simulink model "a_LS_model2"  (R2023b)
settings: Solver=VariableStepAuto  StartTime=0.0  StopTime=3  RelTol=1e-3
PreLoadFcn:
  | %% Model component value calculations with holder values.
  | clear;
  | disp('PreLoaded holder values run model to apply entered T&S values ')
  | 
  | Re = [1, 1]; % The DC resistance of the Voice coil [ohm].
  | 
  | Le = [1, 1]; % The voice coil inductance [H]
  | 
  | Mms = [1, 1]; % Mass of the coil and diaphragm [Kg]
  | 
  | Sd = [1, 1] * 1e-4; % Area of diaphragm [m^2]
  | 
  | Bl = [1, 1]; % The product of magnetic flux density i.e., Force Factor
  | 
  | Vb = [1, 1];
  | 
  | fs = [1, 1];
  | 
  | Qes = [1, 1];
  | 
  | Qms = [1, 1];
  | 
  | Qts = [1, 1];
  | 
  | SweepStart_W_S = 1;
  | SweepEnd_W_S = 1;
  | SweepDuration_W_S = 1;
  | FS = 44100;
  | Qb = 0.707; % Total quality factor
  | 
  | % Constants
  | c = 340; % Speed of sound in m/s
  | rho = 1.2; % Density of air [kg/m^3]
  | r=1; % Distance for farfield calculations
  | wOffset = 0; % Driver offset for fafield calculations
  | tOffset = 0;
  | dt=1/FS; % Time step
  | for n = 1:2
  |     alpha(n) = (Qb^2 - Qts(n)^2) / Qts(n)^2;
  |     Rms(n) = (2 * pi * fs(n) * Mms(n)) / Qms(n);
  |     Cms(n) = 1 / (4 * pi^2 * fs(n)^2 * Mms(n));
  |     Vas(n) = rho * c * Sd(n)^2 * Cms(n);
  | end
  | 
  | QB = sqrt(alpha(1) + 1) * Qts; % Electroacoustics Lecture 4 page 21
  | 
  | for n = 1:2
  |     r = 0.1;
  |     Cab(n) = Vb(n) / (rho * c^2); % Box volume acoustic compliance
  |     a(n) = sqrt(Sd(n) / pi);
  |     a(n) = 0.85;
  | 
  |     % Zc(n) = ((rho * c) / Sd(n)) * c; % from grain42n
  |     Mad(n) = (8 * rho) / (5 * (pi^2) * a(n)); % Mad (acoustic mass)
  |     Mar(n) = rho * ((a(n) * r) / Sd(n)); % from grain42n
  |     Mad(n) = Mar(n);
  | 
  |     Ras(n) = (rho * c) / (pi * (a(n)^2)); % Ras (acoustic resistance), Beranek page 820/ grain42-page 19
  |     Lem(n) = Bl(n)^2 * Cms(n); % Lem (driver's equivalent inductance)
  |     Rem(n) = Bl(n)^2 / Rms(n); % Rem (driver's equivalent mechanical resistance)
  | ... (+17 lines)
StartFcn:
  | %% Model Component Value Calculations
  | close all;
  | 
  | disp('Thiele and Small Parameters Loaded');
  | disp('Loudspeaker Simulation Running...');
  | 
  | % Load parameters from the mask
  | Box_plot_flag = get_param('a_LS_model/T&S Values', 'Box_Plot');
  | Combo_plot_flag = get_param('a_LS_model/T&S Values', 'DSP_Plot');
  | wImpedance_plot_flag = get_param('a_LS_model/T&S Values', 'wImpedance_Plot');
  | tImpedance_plot_flag = get_param('a_LS_model/T&S Values', 'tImpedance_Plot');
  | Re = [str2double(get_param('a_LS_model/T&S Values', 'W_Re')), str2double(get_param('a_LS_model/T&S Values', 'T_Re'))]; % DC resistance of the Voice coil [ohm].
  | Le = [str2double(get_param('a_LS_model/T&S Values', 'W_Le')), str2double(get_param('a_LS_model/T&S Values', 'T_Le'))] * 1e-3; % Voice coil inductance [H]
  | Mms = [str2double(get_param('a_LS_model/T&S Values', 'W_Mms')), str2double(get_param('a_LS_model/T&S Values', 'T_Mms'))] * 1e-3; % Mass of the coil and diaphragm [Kg]
  | Sd = [str2double(get_param('a_LS_model/T&S Values', 'W_Sd')), str2double(get_param('a_LS_model/T&S Values', 'T_Sd'))] * 1e-4; % Area of diaphragm [m^2]
  | Bl = [str2double(get_param('a_LS_model/T&S Values', 'W_Bl')), str2double(get_param('a_LS_model/T&S Values', 'T_Bl'))]; % Magnetic flux density product (Force Factor)
  | Vb = [str2double(get_param('a_LS_model/T&S Values', 'Vb')), str2double(get_param('a_LS_model/T&S Values', 'Vb'))];
  | fs = [str2double(get_param('a_LS_model/T&S Values', 'W_fs')), str2double(get_param('a_LS_model/T&S Values', 'T_fs'))];
  | Cms = [str2double(get_param('a_LS_model/T&S Values', 'W_Cms')), str2double(get_param('a_LS_model/T&S Values', 'W_Cms'))];
  | Qes = [str2double(get_param('a_LS_model/T&S Values', 'W_Qes')), str2double(get_param('a_LS_model/T&S Values', 'T_Qes'))];
  | Qms = [str2double(get_param('a_LS_model/T&S Values', 'W_Qms')), str2double(get_param('a_LS_model/T&S Values', 'T_Qms'))];
  | Qts = [str2double(get_param('a_LS_model/T&S Values', 'W_Qts')), str2double(get_param('a_LS_model/T&S Values', 'T_Qts'))];
  | 
  | % Load additional parameters
  | SweepStart_W_S = str2double(get_param('a_LS_model/Subsystem4', 'SweepStart'));
  | SweepEnd_W_S = str2double(get_param('a_LS_model/Subsystem4', 'SweepStop'));
  | SweepDuration_W_S = str2double(get_param('a_LS_model/Subsystem4', 'SweepTime'));
  | 
  | figSaveFolder = get_param('a_LS_model/Teensy Script', 'figSaveFolder');
  | 
  | FS = 44100;
  | 
  | % Constants
  | c = 343; % Speed of sound in m/s
  | rho = 1.2; % Density of air [kg/m^3]
  | wOffset = str2double(get_param('a_LS_model/Subsystem1', 'distW'));
  | tOffset = str2double(get_param('a_LS_model/Subsystem1', 'distT'));
  | dt=1/FS; %time step
  | 
  | Vas(1) = rho * c * Sd(1)^2 * Cms(1);
  | 
  | for n = 1:2
  |     if n == 1
  |      fsBx = fs(1) *(Vas(1)/Vb(1)+1)^(1/2);
  |      aV = Vas(1) / Vb(1);
  |      Qb(n) = Qts(n) * sqrt(1 + aV);
  |      Rms(n) = (2 * pi * fs(n) * Mms(n)) / Qms(n);
  |      Cms(n) = 1 / ((2 * pi * fs(n))^2 * Mms(n));
  |      CmsBx = 1 / ((2 * pi * fsBx)^2 * Mms(n));
  |      QmsBx =  (2*pi*fsBx*Mms(1))/Rms(1);
  |      RmsBx = (2 * pi * fsBx * Mms(n)) / (QmsBx);
  |     elseif n == 2
  | 
  |      Cms(n) = 1 / ((2 * pi * fs(n))^2 * Mms(n));
  |      Rms(n) = (2 * pi * fs(n) * Mms(n)) / Qms(n);
  |      Vas(n) = rho * c * Sd(n)^2 * Cms(n);
  | 
  |     end
  |    alpha(n) = (Qb^2 - Qts(n)^2) / Qts(n)^2;
  | 
  | ... (+443 lines)
StopFcn:
  | disp('Simulation Ended')
undefined symbols (not defined in the file): Ced, Cem, Cer, Leb, Lem, Rem
libraries: fl_lib x29, nesl_utility x12, dspsrcs4 x1
(part 2 of 2)

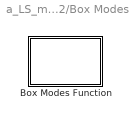
== system a_LS_model2/Box Modes ==
  Box Modes Function : MATLAB Function  TreatAsAtomicUnit=on

== system a_LS_model2/Bypass ==

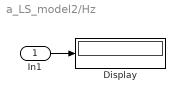
== system a_LS_model2/Hz ==
  In1 : Inport
  Display : Display
  wires:
  In1/1 -> Display/1

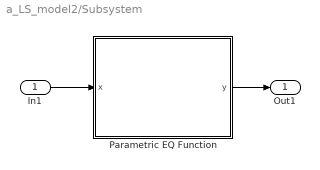
== system a_LS_model2/Subsystem ==
  In1 : Inport
  Parametric EQ Function : MATLAB Function  TreatAsAtomicUnit=on
  Out1 : Outport
  wires:
  In1/1 -> Parametric EQ Function/1(x)
  Parametric EQ Function/1(y) -> Out1/1

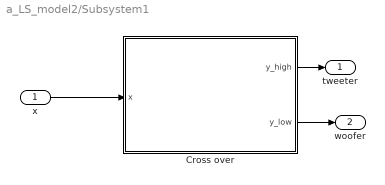
== system a_LS_model2/Subsystem1 ==
  x : Inport
  Cross over : MATLAB Function  TreatAsAtomicUnit=on
  tweeter : Outport
  woofer : Outport  Port=2
  wires:
  x/1 -> Cross over/1(x)
  Cross over/1(y_high) -> tweeter/1
  Cross over/2(y_low) -> woofer/1

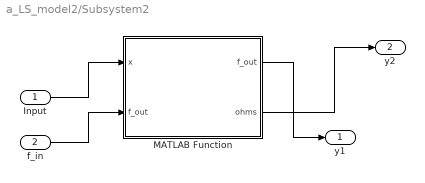
== system a_LS_model2/Subsystem2 ==
  Input : Inport
  f_in : Inport  Port=2
  MATLAB Function : MATLAB Function  TreatAsAtomicUnit=on
  y1 : Outport
  y2 : Outport  Port=2
  wires:
  MATLAB Function/1(f_out) -> y1/1
  Input/1 -> MATLAB Function/1(x)
  MATLAB Function/2(ohms) -> y2/1
  f_in/1 -> MATLAB Function/2("f_out ")

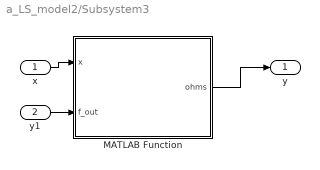
== system a_LS_model2/Subsystem3 ==
  x : Inport
  y1 : Inport  Port=2
  MATLAB Function : MATLAB Function  TreatAsAtomicUnit=on
  y : Outport
  wires:
  x/1 -> MATLAB Function/1(x)
  MATLAB Function/1(ohms) -> y/1
  y1/1 -> MATLAB Function/2(f_out)

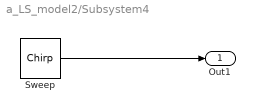
== system a_LS_model2/Subsystem4 ==
  Sweep : dspsrcs4/Chirp  sweep=Logarithmic  mode=Unidirectional  f0=SweepStart  f1=SweepStop  t1=SweepTime  Tsweep=SweepTime  phase=0  Ts=1/FS  spf=1024  datatype=Double  OutputFrames=off
  Out1 : Outport
  wires:
  Sweep/1 -> Out1/1

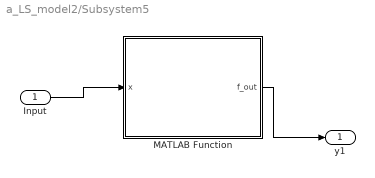
== system a_LS_model2/Subsystem5 ==
  Input : Inport
  MATLAB Function : MATLAB Function  TreatAsAtomicUnit=on
  y1 : Outport
  wires:
  MATLAB Function/1(f_out) -> y1/1
  Input/1 -> MATLAB Function/1(x)

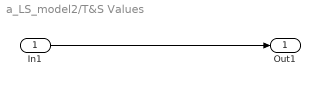
== system a_LS_model2/T&S Values ==
  In1 : Inport
  Out1 : Outport
  wires:
  In1/1 -> Out1/1

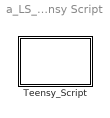
== system a_LS_model2/Teensy Script ==
  Teensy_Script : MATLAB Function  TreatAsAtomicUnit=on

== matlab function a_LS_model2/Subsystem1/Cross over ==
  data: x input; y_high output; y_low output
%% Linkwitz and Riley Crossover function that recieves user parameters from Simulink mask

function [y_high,y_low]= crossover(x)

persistent zi_low_1 % Persistent filter states held over for next block
persistent zi_low_2

persistent zi_high_1
persistent zi_high_2



persistent flagBaseAssign             % flags for parts of code that only need to be run once to improve code efficiency



persistent frontPadT
persistent frontPadW
persistent delayBufferT
persistent delayBufferW


if isempty(flagBaseAssign)

    flagBaseAssign=1;

end


%wSamples=double(0);
%tSamples=double(0);
coder.extrinsic('get_param') %coder.entrinsic allows for functions to be surported in simulink that would otherwise not be
coder.extrinsic('xticks')
coder.extrinsic('xticklabels')
coder.extrinsic("assignin")
coder.extrinsic("evalin")
coder.extrinsic("sgtitle")
coder.extrinsic("cat")
coder.extrinsic("exist")
coder.extrinsic("mkdir")
coder.extrinsic("fullfile")
coder.extrinsic("mexFilter")




y_low =zeros(length(x),1);
y_high=zeros(length(x),1);


%Getting user input from mask

persistent tDistance wDistance G_T G_W filterOrder delayInfo B_low A_low B_high A_high plotFlag bypass fs...
    tweeterGain_dB wooferGain_dB

if isempty (tDistance)
    plotFlag = get_param('a_LS_model/Subsystem1', 'response');
    bypass = get_param('a_LS_model/Bypass', 'bypass');
    fs=44100;
    tDistance=double(0);
    tDistance = str2double(get_param('a_LS_model/Subsystem1', 'distT'));
    wDistance=double(0);
    wDistance = str2double(get_param('a_LS_model/Subsystem1', 'distW'));
    

    G_T = str2double(get_param('a_LS_model/Subsystem1', 'G_T'));
    G_W = str2double(get_param('a_LS_model/Subsystem1', 'G_W'));
    filterOrder = get_param('a_LS_model/Subsystem1', 'filter_order');
    delayInfo = get_param('a_LS_model/Subsystem1', 'delay');
    tweeterGain_dB = (10^(G_T/20));
    wooferGain_dB = (10^(G_W/20));

    fc = str2double(get_param('a_LS_model/Subsystem1', 'fc'));


    w=double(0);

    w =fc/(fs/2);



    if strcmp(filterOrder,'8th')

        butterOrder=4;

    elseif strcmp(filterOrder,'4th')

        butterOrder=2;

    else

        butterOrder=1;
    end



    [B_low, A_low]= butter(butterOrder, w, "low");

    [B_high, A_high]= butter(butterOrder, w, "high");



    assignin('base', 'B_Low_shel', B_low); % Assign to base for use in teensy script writing also speeds code as can be read rather than calulated for every block but first.
    assignin('base', 'A_Low_shel', A_low);

    assignin('base', 'B_High_shel', B_high);
    assignin('base', 'A_High_shel', A_high);





end


%%%%%%%%%%%%%%%%%%%%%%%%%%%%%%%%%%%%%%%%%%%%%%%%%%%%%%%%%%%%%%%%%%%%%%
%% Low pass


x_low=x;

if isempty (zi_low_1)
    zi_low_1=zeros(5,1);
    zi_low_2=zeros(5,1);


    zi_high_1=zeros(5,1);
    zi_high_2=zeros(5,1);

end




[y_low, zi_low_1]=mexFilter(B_low, A_low,x_low, zi_low_1);


x_low =y_low;

[y_low, zi_low_2]=mexFilter(B_low, A_low, x_low, zi_low_2);










%%%%%%%%%%%%%%%%%%%%%%%%%%%%%%%%%%%%%%%%%%%%%%%%%%%%%%%%%%%%%%%
%% High pass


x_high=x;



[y_high, zi_high_1]=mexFilter(B_high,A_high,x_high,zi_high_1);

x_high=y_high;


[y_high, zi_high_2]=mexFilter(B_high,A_high,x_high,zi_high_2);



y_high=y_high * tweeterGain_dB;
y_low=y_low * wooferGain_dB;


y_checkLow=y_low;   %%For delay debugging
y_checkHigh=y_high;


%% Plotting

if strcmp(plotFlag,'on')
    figure(2)

    [H_high, ~]=freqz(B_high,A_high);
    [H_low, w]=freqz(B_low,A_low);


    f=w/(2*pi)*fs;

    H_high_2=H_high.*H_high;

    H_low_2=H_low.*H_low;


    set(gcf, 'Position', [100, 100, 800, 600]);

    [H_high, ~]=freqz(B_high,A_high);
    [H_low, w]=freqz(B_low,A_low);


    f=w/(2*pi)*fs;

    H_high_2=H_high.*H_high;

    H_low_2=H_low.*H_low;



    subplot(3,1,1)
    semilogx(f, mag2db(abs(H_high_2)),'b-','DisplayName', 'Second Cascade');
    hold on
    semilogx(f, mag2db(abs(H_high)),'g-', 'DisplayName', 'First Cascade');
    hold off
    xlabel('Frequency (Hz)')
    ylabel('Magnitude (dB)')
    title('Magnitude Response High Pass')
    ylim([-14 14])
    xlim([min(f) max(f)])

    xticks([20 50 100 200 500 1000 2000 5000 10000 20000]);
    xticklabels({'20','50','100','200','500','1000','2000','5000','10000','20000'});
    legend('show', 'Location', 'best');
    subplot(3,1,2)
    semilogx(f, mag2db(abs(H_low_2)),'b-','DisplayName', 'Second Cascade');
    hold on
    semilogx(f, mag2db(abs(H_low)),'g-','DisplayName', 'First Cascade');
    hold off
    xlabel('Frequency (Hz)')
    ylabel('Magnitude (dB)')
    title('Magnitude Response Low pass')
    ylim([-14 14])
    xlim([min(f) max(f)])

    xticks([20 50 100 200 500 1000 2000 5000 10000 20000]);
    xticklabels({'20','50','100','200','500','1000','2000','5000','10000','20000'});
    legend('show', 'Location', 'best');
    subplot(3,1,3)
    semilogx(f, mag2db(abs(H_low_2)),'r--','DisplayName', 'Low Pass');
    hold on
    semilogx(f, mag2db(abs(H_high_2)),'r-','DisplayName', 'High Pass');
    legend('show', 'Location', 'best');
    if double(length(B_low))==2

        H_low_2_inverted=H_low_2.*-1;
        semilogx(f, mag2db(abs(H_high_2+H_low_2_inverted)),'b-','DisplayName', 'Combined Response');


        hold off
        xlabel('Frequency (Hz)')
        ylabel('Magnitude (dB)')
        title('Magnitude Response Linkwitz-Riley 2nd Order')

    elseif double(length(B_low))==3

        semilogx(f, mag2db(abs(H_high_2+H_low_2)),'b-','DisplayName', 'Combined Response');


        hold off
        xlabel('Frequency (Hz)')
        ylabel('Magnitude (dB)')
        title('Magnitude Response Linkwitz-Riley 4th Order')


    else

        semilogx(f, mag2db(abs(H_high_2+H_low_2)),'b-','DisplayName', 'Combined Response');


        hold off
        xlabel('Frequency (Hz)')
        ylabel('Magnitude (dB)')
        title('Magnitude Response Linkwitz-Riley 8th Order')

    end


    ylim([-14 14])
    xlim([min(f) max(f)])

    xticks([20 50 100 200 500 1000 2000 5000 10000 20000]);
    xticklabels({'20','50','100','200','500','1000','2000','5000','10000','20000'});

    if strcmp(filterOrder,'4th')

        sgtitle('Linkwitz-Riley 4th Order Crossover');

    elseif strcmp(filterOrder,'8th')

        sgtitle('Linkwitz-Riley 8th Order Crossover');

    else

        sgtitle('Linkwitz-Riley 2nd Order Crossover');

    end
    if strcmp(get_param('a_LS_model/Teensy Script', 'saveFigs'),"on")

        figSaveFolder = get_param('a_LS_model/Teensy Script', 'figSaveFolder');

        if ~exist(figSaveFolder, 'dir')

            mkdir(figSaveFolder);

        end




        saveas(gcf,fullfile(figSaveFolder,[figSaveFolder,'_crossOver.png']));
    end
    plotFlag = 'off';



end



%% Tweeter Delay

if wDistance>0 %%if woofer has been offset (back) delay sound to tweeter by the appropriate amount

    

    y_high_Delayed = zeros(length(x),1);


    if flagBaseAssign==1
        tSamplesInM = double(0);%samples in meters
        tSamples = double(0);
        C = double(343);
        tSamplesInM = (fs / C);
        tSamples = round(tSamplesInM * wDistance);
        assignin('base', 'tSamples', tSamples);


    else

        tSamples=evalin('base', 'tSamples');



    end

    if isempty(frontPadT)
        frontPadT = zeros(tSamples, 1);
        delayBufferT = y_high(end - tSamples + 1:end);
    else
        frontPadT = delayBufferT;
    end



    y_high_Delayed(1:end) = [frontPadT; y_high(1:end - tSamples)];

    delayBufferT = y_high(end - tSamples + 1:end);

    y_high=y_high_Delayed;


else
    assignin('base', 'tSamples', 0);

end






%% Woofer Delay

if tDistance>0 %%if tweeter has been offset (back) delay sound to woofer by the appropriate amount


    y_low_Delayed = zeros(length(x),1);



    if flagBaseAssign==1

        wSamplesInM = double(0);
        wSamples = double(0);
        C = double(343);
        wSamplesInM = (fs / C);
        wSamples = round(wSamplesInM * tDistance);
        assignin('base', 'wSamples', wSamples);




    else

        wSamples=evalin('base', 'wSamples');


    end



    if isempty(frontPadW)

        frontPadW = zeros(wSamples, 1);
        delayBufferW = y_low(end - wSamples + 1:end);

    else

        frontPadW = delayBufferW;

    end




    y_low_Delayed(1:end) = [frontPadW; y_low(1:end - wSamples)];

    delayBufferW = y_low(end - wSamples + 1:end);

    y_low=y_low_Delayed;

else
    assignin('base', 'wSamples', 0);

end

if strcmp(delayInfo, 'on')



    if (flagBaseAssign==1)

        figure(7)

        subplot(2,1,1)

        plot(y_checkLow, '-', 'LineWidth', 1, 'DisplayName', 'Woofer')
        hold on;
        plot(y_low, '-', 'LineWidth', 1, 'DisplayName', 'Woofer Delayed');
        hold off
        legend('show');
        xlabel('Samples')
        ylabel('Amplitude')
        title("Woofer Delay")



        subplot(2,1,2)

        plot(y_checkHigh, '-', 'LineWidth', 1,  'DisplayName', 'Tweeter ');
        hold on
        plot(y_high, '-', 'LineWidth', 1,  'DisplayName', 'Tweeter Delayed');
        hold off
        legend('show');
        title("Tweeter Delay")
        xlabel('Samples')
        ylabel('Amplitude')
        if strcmp(get_param('a_LS_model/Teensy Script', 'saveFigs'),"on")
            figSaveFolder = get_param('a_LS_model/Teensy Script', 'figSaveFolder');
            saveas(gcf,fullfile(figSaveFolder,[figSaveFolder,'_delay.png']));
        end
    end



end



if strcmp(filterOrder,'2nd')

    y_low=y_low.*-1; %inverse phase for 2nd order L&R

end

if (flagBaseAssign == 1)

    flagBaseAssign=2;

end



if strcmp('on',bypass)%not strictly a bypass but done like this so variables are still created and assigned for the sccript generation

    y_high=x;
    y_low = x;


end

end








%%%%%%%%%%%%%%%%%%%%%%%%%%%%%%%%%%%%%%%%%%%%%
%% filter function

function [y, zf] = TDF2Filter(B, A, x,zi)




b0=double(B(1));
b1=double(B(2));


a0=double(A(1));
a1=double(A(2));


xLength = length(x);
if length(B)==3

    b2=double(B(3));
    a2=double(A(3));
    
    
    y = ones(length(x),1);
    
        for n = 1:xLength
            
        
            y(n) = (b0/a0) * x(n) + zi(1);
            
            zi(1) = (b1/a0) * x(n) + zi(2) - (a1/a0) * y(n);
           
           
             zi(2) = (b2/a0) * x(n) + zi(3) - (a2/a0) * y(n);
            
      
        end


elseif length(B)==5


    b2=(B(3));
    a2=(A(3));
    b3=(B(4));
    a3=(A(4));
    b4=(B(5));
    a4=(A(5));


    
    
    y = ones(xLength,1);
    
        for n = 1:xLength
            
        
            y(n) = (b0/a0) * x(n) + zi(1);
            
            zi(1) = (b1/a0) * x(n) + zi(2) - (a1/a0) * y(n);
           
           
             zi(2) = (b2/a0) * x(n) + zi(3) - (a2/a0) * y(n);
        
             zi(3) = (b3/a0) * x(n) + zi(4) - (a3/a0) * y(n);
        
             zi(4) = (b4/a0) * x(n) + zi(5) - (a4/a0) * y(n);
        
  
        end

else

    y = ones(xLength,1);

    for n = 1:xLength
    

        y(n) = (b0/a0) * x(n) + zi(1);
    
        zi(1) = (b1/a0) * x(n) + zi(2) - (a1/a0) * y(n);
    


    end
end

zf = zi;

end

== matlab function a_LS_model2/Subsystem/Parametric EQ Function ==
  data: x input; y output

function y=paramFunc(x)

coder.extrinsic('get_param')
coder.extrinsic('xticks')
coder.extrinsic('xticklabels')
coder.extrinsic('assignin')
coder.extrinsic('evalin')
coder.extrinsic("sgtitle")
coder.extrinsic("exist")
coder.extrinsic("mkdir")
coder.extrinsic("fullfile")
coder.extrinsic("mexFilter")
coder.extrinsic("mexParaFilter")

persistent zi_Arr
persistent plotFlag






%%
%%%%%%%%%%%%%%%%%%%%%%%%%%%%%%%%%%%%%%%%%%%%%%%%%%%%%%%%%%%%%%%%%%%%%%%%%%%%%%%%%%%%%%%%%%%%%%%%%%%%%%%%%%%%%%%%%%%%%%%%%%%%%%%%%%%%





persistent V0 K fc BWp BW N w0 gain Numband V0_peq B A fs

if isempty(gain)
    fs=44100;
    Numband=double(6);
    V0=zeros(Numband,1);
    V0_peq=zeros(Numband,1);
    K= zeros(Numband,1);
    fc=zeros(Numband,1);
    BWp=zeros(Numband,1);
    BW=zeros(Numband,1);
    N=zeros(Numband,1);
    w0=zeros(Numband,1);
    gain= zeros(Numband,1);


    plotFlag = get_param('a_LS_model/Subsystem', 'plotFlag');


    gain(1) = str2double(get_param('a_LS_model/Subsystem', 'GdB1'));
    gain(2) = str2double(get_param('a_LS_model/Subsystem', 'GdB2'));
    gain(3) = str2double(get_param('a_LS_model/Subsystem', 'GdB3'));
    gain(4) = str2double(get_param('a_LS_model/Subsystem', 'GdB4'));
    gain(5) = str2double(get_param('a_LS_model/Subsystem', 'GdB5'));
    gain(6) = str2double(get_param('a_LS_model/Subsystem', 'GdB6'));



    fc(1) = str2double(get_param('a_LS_model/Subsystem', 'FC1'));
    fc(2) = str2double(get_param('a_LS_model/Subsystem', 'FC2'));
    fc(3) = str2double(get_param('a_LS_model/Subsystem', 'FC3'));
    fc(4) = str2double(get_param('a_LS_model/Subsystem', 'FC4'));
    fc(5) = str2double(get_param('a_LS_model/Subsystem', 'FC5'));
    fc(6) = str2double(get_param('a_LS_model/Subsystem', 'FC6'));


    BWp(1) = str2double(get_param('a_LS_model/Subsystem', 'BW1'));
    BWp(2) = str2double(get_param('a_LS_model/Subsystem', 'BW2'));
    BWp(3) = str2double(get_param('a_LS_model/Subsystem', 'BW3'));
    BWp(4) = str2double(get_param('a_LS_model/Subsystem', 'BW4'));
    BWp(5) = str2double(get_param('a_LS_model/Subsystem', 'BW5'));
    BWp(6) = str2double(get_param('a_LS_model/Subsystem', 'BW6'));

    Filt=zeros(Numband,4);
    b0=double(0);
    b1=double(0);
    b2=double(0);
    a0=double(0);
    a1=double(0);
    a2=double(0);

    for i=1:Numband

        Filt(i,1)= gain(i);
        Filt(i,2)=fc(i);
        Filt(i,3)=BWp(i);
        Filt(i,4)=BWp(i)*gain(i);
    end

    minFc=min(Filt(1:end,2));
    maxFc=max(Filt(1:end,2));



    for i=1:Numband
        V0(i)= 10^(Filt(i,1)/20);%For shelving filters
        K(i)= tan ((pi*fc(i))/fs);

        V0_peq(i)=Filt(i,1);%For peaking filter
        w0(i) = Filt(i,2)/(fs/2);
        N=double(2);


        y=zeros(length(x),1);

        BW(i)=(Filt(i,2)*Filt(i,3))/100;%percentage of fc to Hz
        BW(i)=BW(i)/(fs/2);

    end

    [B,A] = designParamEQ(2,V0_peq',w0', BW','Orientation','row');



    for i=1:Numband


        if Filt(i,2) ==minFc && V0(i)>0
            %Low Shelf Boost
            b0 = ((1)+(sqrt(2*V0(i))*K(i))+V0(i)*K(i)^2) / ((1)+(sqrt(2)*K(i))+K(i)^2);
            b1 = ((2)*(V0(i)*(K(i)^2)-1)) / ((1)+(sqrt(2)*K(i))+K(i)^2);
            b2 = ((1)-(sqrt(2*V0(i))*K(i))+V0(i)*K(i)^2) / ((1)+(sqrt(2)*K(i))+K(i)^2);
            a0 = 1;
            a1 =  ((2)*((K(i)^2)-1)) / ((1)+(sqrt(2)*K(i))+K(i)^2);
            a2 = ((1)-sqrt(2)*K(i)+K(i)^2) / ((1)+(sqrt(2)*K(i))+K(i)^2);

            B(i,:)=[b0,b1,b2];
            A(i,:)=[a0,a1,a2];


        elseif Filt(i,2) == minFc && V0(i)<0
            %Low Shelf Cut


            b0=(V0(i)*(1+sqrt(2)*K(i)+K(i)^2)) / (V0(i)+sqrt(2*V0(i))*K(i)+K(i)^2);
            b1=(2*V0(i)*(K(i)^2-1)) / (V0(i)+sqrt(2*V0(i))*K(i)+K(i)^2);
            b2=(V0(i)*(1-sqrt(2)*K(i)+K(i)^2)) / (V0(i)+sqrt(2*V0(i))*K(i)+K(i)^2);
            a0=1;
            a1=(2*(K(i)^2-V0(i))) / (V0(i)+sqrt(2*V0(i))*K(i)+K(i)^2);
            a2=(V0(i)-sqrt(2*V0(i))*K(i)+K(i)^2) / (V0(i)+sqrt(2*V0(i))*K(i)+K(i)^2);

            B(i,:)=[b0,b1,b2];
            A(i,:)=[a0,a1,a2];


        elseif Filt(i,2) ==maxFc && V0(i)>0
            % High Shelf Boost
            b0 = (V0(i)+sqrt(2*V0(i))*K(i)+K(i)^2) /(1+sqrt(2)*K(i)+K(i)^2);
            b1= (2*(K(i)^2-V0(i))) / (1+sqrt(2)*K(i)+K(i)^2);
            b2=  (V0(i)-sqrt(2*V0(i))*K(i)+K(i)^2) / (1+sqrt(2)*K(i)+K(i)^2);
            a0=1;
            a1= (2*(K(i)^2-1)) / (1+(sqrt(2)*K(i))+K(i)^2);
            a2= (1-(sqrt(2)*K(i))+K(i)^2) / (1+(sqrt(2)*K(i))+K(i)^2);

            B(i,:)=[b0,b1,b2];
            A(i,:)=[a0,a1,a2];



        elseif Filt(i,2) == maxFc && V0(i)<0
            %High Shelf Cut

            b0=(V0(i)*(1+sqrt(2)*K(i)+K(i)^2)) / (1+sqrt(2*V0(i))*K(i)+V0(i)*K(i)^2);
            b1=(2*V0(i)*(K(i)^2-1)) / (1+sqrt(2*V0(i))*K(i)+V0(i)*K(i)^2);
            b2=(V0(i)*(1-sqrt(2)*K(i)+K(i)^2)) / (1+sqrt(2*V0(i))*K(i)+V0(i)*K(i)^2);
            a0=1;
            a1=(2*(V0(i)*K(i)^2-1)) / (1+sqrt(2*V0(i))*K(i)+V0(i)*K(i)^2);
            a2=(1-sqrt(2*V0(i))*K(i)+V0(i)*K(i)^2) / (1+sqrt(2*V0(i))*K(i)+V0(i)*K(i)^2);



            B(i,:)=[b0,b1,b2];
            A(i,:)=[a0,a1,a2];



        end

    end

    assignin('base', 'B_paramet', B);
    assignin('base', 'A_paramet', A);
  



end

%%
%%%%%%%%%%%%%%%%%%%%%%%%%%%%%%%%%%%%%%%%%%%%%%%%%%%%%%%%%%%%%%%%%%%%%%%%%%%%%%%%%%%%%%%%%%%%%%%%%%%%%%%%%%%%%%%%%%%%%%%%%

if isempty(zi_Arr)
    zi_Arr=zeros(3,Numband);
end


for n=1:6


    [y, zi_Arr(:,n)]=mexParaFilter(B(n,:),A(n,:),x,zi_Arr(:,n));

    x=y;



    %%
    %%%%%%%%%%%%%%%%%%%%%%%%%%%%%%%%%%%%%%%%%%%%%%%%%%%%%%%%%%%%%%%%%%%%%%%%%%%%%%%%%%%%%%%%%%%%%%%%%%%%%%%%%%%%%%%%%%%%%%%


end

if strcmp(plotFlag, 'on')

    zeroLine = zeros(512,1);
    H=complex(ones(512,1));
    H_temp=complex(ones(512,Numband));


    for n=1:Numband
        [H_temp(1:end,n),w] = freqz(B(n,1:end),A(n,1:end));

        H=H.*H_temp(1:end,n);

        f=w/(2*pi)*fs;

        if n==Numband 
            assignin('base', 'H_Vector', mag2db(abs(H)));
            assignin('base', 'F_Vector', f);
        
            figure(1)
            subplot(2,1,1)
            assignin('base', 'H_Vector', mag2db(abs(H)));
            assignin('base', 'F_Vector', f);
            semilogx(f, zeroLine,'Color','#d3d3d3');
            hold on
            semilogx(f, mag2db(abs(H)));

            hold off
            xlabel('Frequency (Hz)')
            ylabel('Magnitude (dB)')
            title('Magnitude Response')
            ylim([-4 4])
            xlim([min(f) max(f)])

            xticks([20 50 100 200 500 1000 2000 5000 10000 20000]);
            xticklabels({'20','50','100','200','500','1000','2000','5000','10000','20000'});

            subplot(2,1,2)
            plot(w, angle(H));
            xlabel('Normalized Frequency (rad/sample)')
            ylabel('Phase (rad)')
            title('Phase Response')


            plotFlag = 'off';
            sgtitle('Parametric EQ');
            if strcmp(get_param('a_LS_model/Teensy Script', 'saveFigs'),"on")

                figSaveFolder = get_param('a_LS_model/Teensy Script', 'figSaveFolder');


                if ~exist(figSaveFolder, 'dir')

                    mkdir(figSaveFolder);

                end

                saveas(gcf,fullfile(figSaveFolder,[figSaveFolder,'_parametric.png']));

            end

        end
    end


end


end
%%
%%%%%%%%%%%%%%%%%%%%%%%%%%%%%%%%%%%%%%%%%%%%%%%%%%%%%%%%%%%%%%%%%%%%%%%%%%%%%%%%%%%%%%%%%%%%%%%%%%%%%%%%%%%%%%%%%%%%%%%%%%%%%%%%%%%%%%%55

function [y, zf] = TDF2Filter(B, A, x, zi)




b0=B(1);
b1=B(2);
b2=B(3);
a0=A(1);
a1=A(2);
a2=A(3);

xLength = length(x);
y = ones(xLength, 1);

for n = 1:xLength
    

    y(n) = (b0/a0) * x(n) + zi(1);
    
    zi(1) = (b1/a0) * x(n) + zi(2) - (a1/a0) * y(n);
   
    zi(2) = (b2/a0) * x(n) + zi(3) - (a2/a0) * y(n);
    

end



zf = zi;

end

== matlab function a_LS_model2/Subsystem2/MATLAB Function ==
  data: f_out output; x input; f_out input; ohms output

function [f_out, ohms]=variableResistor(x, f_out)

coder.extrinsic('get_param')
coder.extrinsic('ohmsCalc')



persistent rho c Sd Bl fs r Zc 




if isempty(Sd)
    
    Sd= str2double(get_param('a_LS_model/T&S Values', 'W_Sd'))    *1e-4;  %Area of diagphram [m^2]
    Bl= str2double(get_param('a_LS_model/T&S Values', 'W_Bl'));            %The product of magnetic flux density ie Force Factor

    c=344;% speed of sound m/s
    rho=1.2;% density of air [kg/m^3]
    Zc=(rho*c/Sd)*c;
    r=sqrt(Sd/pi);
    fs=44100;

    ohms=zeros(size(x));
  

end
tic

ohms = ohmsCalc(f_out, fs, r, Zc, Bl, Sd);


% w=2*pi*f_out/fs;
% k=w/c;
% 
% Rar=Zc*(1/4)*(k*r).^2;
% Rer=((Bl/Sd)^2)*(1./Rar);
%  
% ohms=Rer;




%%
%%%%%%%%%%%%%%%%%%%%%%%%%%%%%%%%%%%%%%%%%%%%%%%%%%%%%%%%%%%%%%%%%%%%%%%%%%%%%%%%%%%%%%%%%%%%%%%%%%%%%%%%%%%%%%%%%%%%%%%%%%%%%%%%%%%%





end

== matlab function a_LS_model2/Subsystem3/MATLAB Function ==
  data: x input; ohms output; f_out input

function ohms  =variableResistor(x, f_out)

coder.extrinsic('get_param')
coder.extrinsic('ohmsCalc')





persistent rho c Sd Bl  fs r Zc




if isempty(Sd)

    Sd= str2double(get_param('a_LS_model/T&S Values', 'T_Sd'))    *1e-4;  %Area of diagphram [m^2]
    Bl= str2double(get_param('a_LS_model/T&S Values', 'T_Bl'));            %The product of magnetic flux density ie Force Factor

    c=344;% speed of sound m/s
    rho=1.2;% density of air [kg/m^3]
    Zc=(rho*c/Sd)*c;
    r=sqrt(Sd/pi);
    fs=44100;
    ohms=zeros(size(x));

end


ohms = ohmsCalc(f_out, fs, r, Zc, Bl, Sd);

% w=2*pi*f_out/fs;
% 
% 
% k=w/c;
% 
% Rar=Zc*(1/4)*(k*r).^2;
% Rer=((Bl/Sd)^2)*(1./Rar);
% 
% 
% ohms=Rer;




%%
%%%%%%%%%%%%%%%%%%%%%%%%%%%%%%%%%%%%%%%%%%%%%%%%%%%%%%%%%%%%%%%%%%%%%%%%%%%%%%%%%%%%%%%%%%%%%%%%%%%%%%%%%%%%%%%%%%%%%%%%%%%%%%%%%%%%





end

== matlab function a_LS_model2/Teensy Script/Teensy_Script ==
%% Creates an arduino script that the user copies into the Teensy SDK



function teensyScriptGen

persistent flag

coder.extrinsic('get_param') %coder.entrinsic allows for functions to be surported in simulink that would otherwise not be
coder.extrinsic('evalin')
coder.extrinsic('datestr')
coder.extrinsic('copyfile')


saveName = get_param('a_LS_model/Teensy Script', 'savename'); %gets save name for script from mask
nanExpected = 72;
if isempty(flag) % Script runs just once flag
    flag=1;
end

if flag==1
    
    fc = str2double(get_param('a_LS_model/Subsystem1', 'fc'));
    filterOrder = get_param('a_LS_model/Subsystem1', 'filter_order'); 
    tDistance = str2double(get_param('a_LS_model/Subsystem1', 'distT'));
    wDistance = str2double(get_param('a_LS_model/Subsystem1', 'distW'));
    tSamples = evalin('base', 'tSamples'); 
    wSamples = evalin('base', 'wSamples'); 
    gainW = str2double(get_param('a_LS_model/Subsystem1', 'G_W'));
    gainT = str2double(get_param('a_LS_model/Subsystem1', 'G_T'));
    A_paramet = evalin('base', 'A_paramet');
    B_paramet = evalin('base', 'B_paramet');

    A_Hi = evalin('base', 'A_High_shel');
    A_Lo = evalin('base', 'A_Low_shel');

    B_Hi = evalin('base', 'B_High_shel');
    B_Lo = evalin('base', 'B_Low_shel');


    if strcmp(filterOrder,'4th')
        
        B_Lo_Length=int16(3);

    elseif strcmp(filterOrder,'8th')

        B_Lo_Length=int16(5);

    else

        B_Lo_Length=int16(2);
    end



  a0_1=A_paramet(1,1); a1_1=A_paramet(1,2); a2_1=A_paramet(1,3) ; b0_1=B_paramet(1,1) ; b1_1=B_paramet(1,2) ; b2_1=B_paramet(1,3) ;
  a0_2=A_paramet(2,1) ; a1_2=A_paramet(2,2) ; a2_2=A_paramet(2,3) ; b0_2=B_paramet(2,1) ; b1_2=B_paramet(2,2) ; b2_2=B_paramet(2,3) ;
  a0_3=A_paramet(3,1) ; a1_3=A_paramet(3,2) ; a2_3=A_paramet(3,3) ; b0_3=B_paramet(3,1) ; b1_3=B_paramet(3,2) ; b2_3=B_paramet(3,3) ;
  a0_4=A_paramet(4,1) ; a1_4=A_paramet(4,2) ; a2_4=A_paramet(4,3) ; b0_4=B_paramet(4,1) ; b1_4=B_paramet(4,2) ; b2_4=B_paramet(4,3) ;
  a0_5=A_paramet(5,1); a1_5=A_paramet(5,2) ; a2_5=A_paramet(5,3) ; b0_5=B_paramet(5,1) ; b1_5=B_paramet(5,2) ; b2_5=B_paramet(5,3) ;
  a0_6=A_paramet(6,1) ; a1_6=A_paramet(6,2) ; a2_6=A_paramet(6,3) ; b0_6=B_paramet(6,1) ; b1_6=B_paramet(6,2) ; b2_6=B_paramet(6,3) ;
  
 
  a0_Lo=A_Lo(1,1) ; a1_Lo=A_Lo(1,2); b0_Lo=B_Lo(1,1)  ; b1_Lo=B_Lo(1,2) ; 
  a0_Hi=A_Hi(1,1); a1_Hi=A_Hi(1,2) ;b0_Hi=B_Hi(1,1);   b1_Hi=B_Hi(1,2); 
  


% Load script template, this needs to be in the same root as simulink
% model
fileID = fopen('script_template.txt', 'r');
if fileID == -1
    error('Error: Could not open script_template.txt. Check if the file is in the root folder.');
else
originalScript = char(fread(fileID, '*char')');
fclose(fileID);
end
nanCounted = int16(count(originalScript, ' nan'));
if (nanExpected~= nanCounted)
    sprintf("ERROR. Template check failed. Expected %d nan, found:", nanExpected);
    disp(nanCounted)%% This is just some error mitigation as I kept overwriting the nan values while making edits and not noticing 
else
    disp("Template check passed")
end


% Replace NaN values 
d = datestr(datetime('now'));
tempScript = strrep(originalScript, 'Script generated: nan', sprintf('Script generated: "%s";', d));
tempScript = strrep(tempScript, 'a0_1 = nan', sprintf('a0_1 = %.31f', a0_1)); 
tempScript = strrep(tempScript, 'a1_1 = nan', sprintf('a1_1 = %.31f', a1_1));
tempScript = strrep(tempScript, 'a2_1 = nan', sprintf('a2_1 = %.31f', a2_1));
tempScript = strrep(tempScript, 'b0_1 = nan', sprintf('b0_1 = %.31f', b0_1));
tempScript = strrep(tempScript, 'b1_1 = nan', sprintf('b1_1 = %.31f', b1_1));
tempScript = strrep(tempScript, 'b2_1 = nan', sprintf('b2_1 = %.31f', b2_1));



tempScript = strrep(tempScript, 'a0_2 = nan', sprintf('a0_2 = %.31f', a0_2));
tempScript = strrep(tempScript, 'a1_2 = nan', sprintf('a1_2 = %.31f', a1_2));
tempScript = strrep(tempScript, 'a2_2 = nan', sprintf('a2_2 = %.31f', a2_2));
tempScript = strrep(tempScript, 'b0_2 = nan', sprintf('b0_2 = %.31f', b0_2));
tempScript = strrep(tempScript, 'b1_2 = nan', sprintf('b1_2 = %.31f', b1_2));
tempScript = strrep(tempScript, 'b2_2 = nan', sprintf('b2_2 = %.31f', b2_2));



tempScript = strrep(tempScript, 'a0_3 = nan', sprintf('a0_3 = %.31f', a0_3));
tempScript = strrep(tempScript, 'a1_3 = nan', sprintf('a1_3 = %.31f', a1_3));
tempScript = strrep(tempScript, 'a2_3 = nan', sprintf('a2_3 = %.31f', a2_3));
tempScript = strrep(tempScript, 'b0_3 = nan', sprintf('b0_3 = %.31f', b0_3));
tempScript = strrep(tempScript, 'b1_3 = nan', sprintf('b1_3 = %.31f', b1_3));
tempScript = strrep(tempScript, 'b2_3 = nan', sprintf('b2_3 = %.31f', b2_3));

tempScript = strrep(tempScript, 'a0_4 = nan', sprintf('a0_4 = %.31f', a0_4));
tempScript = strrep(tempScript, 'a1_4 = nan', sprintf('a1_4 = %.31f', a1_4));
tempScript = strrep(tempScript, 'a2_4 = nan', sprintf('a2_4 = %.31f', a2_4));
tempScript = strrep(tempScript, 'b0_4 = nan', sprintf('b0_4 = %.31f', b0_4));
tempScript = strrep(tempScript, 'b1_4 = nan', sprintf('b1_4 = %.31f', b1_4));
tempScript = strrep(tempScript, 'b2_4 = nan', sprintf('b2_4 = %.31f', b2_4));

tempScript = strrep(tempScript, 'a0_5 = nan', sprintf('a0_5 = %.31f', a0_5));
tempScript = strrep(tempScript, 'a1_5 = nan', sprintf('a1_5 = %.31f', a1_5));
tempScript = strrep(tempScript, 'a2_5 = nan', sprintf('a2_5 = %.31f', a2_5));
tempScript = strrep(tempScript, 'b0_5 = nan', sprintf('b0_5 = %.31f', b0_5));
tempScript = strrep(tempScript, 'b1_5 = nan', sprintf('b1_5 = %.31f', b1_5));
tempScript = strrep(tempScript, 'b2_5 = nan', sprintf('b2_5 = %.31f', b2_5));

tempScript = strrep(tempScript, 'a0_6 = nan', sprintf('a0_6 = %.31f', a0_6));
tempScript = strrep(tempScript, 'a1_6 = nan', sprintf('a1_6 = %.31f', a1_6));
tempScript = strrep(tempScript, 'a2_6 = nan', sprintf('a2_6 = %.31f', a2_6));
tempScript = strrep(tempScript, 'b0_6 = nan', sprintf('b0_6 = %.31f', b0_6));
tempScript = strrep(tempScript, 'b1_6 = nan', sprintf('b1_6 = %.31f', b1_6));
tempScript = strrep(tempScript, 'b2_6 = nan', sprintf('b2_6 = %.31f', b2_6));

tempScript = strrep(tempScript, 'a0_Lo = nan', sprintf('a0_Lo = %.31f', a0_Lo));
tempScript = strrep(tempScript, 'a1_Lo = nan', sprintf('a1_Lo = %.31f', a1_Lo));


tempScript = strrep(tempScript, 'b0_Lo = nan', sprintf('b0_Lo = %.31f', b0_Lo));
tempScript = strrep(tempScript, 'b1_Lo = nan', sprintf('b1_Lo = %.31f', b1_Lo));


tempScript = strrep(tempScript, 'a0_Hi = nan', sprintf('a0_Hi = %.31f', a0_Hi));
tempScript = strrep(tempScript, 'a1_Hi = nan', sprintf('a1_Hi = %.31f', a1_Hi));

tempScript = strrep(tempScript, 'b0_Hi = nan', sprintf('b0_Hi = %.31f', b0_Hi));
tempScript = strrep(tempScript, 'b1_Hi = nan', sprintf('b1_Hi = %.31f', b1_Hi));


tempScript = strrep(tempScript, 'B_Lo_Length = nan', sprintf('B_Lo_Length = %d', B_Lo_Length));

tempScript = strrep(tempScript, 'tSamples = nan', sprintf('tSamples = %d', tSamples));
tempScript = strrep(tempScript, 'wSamples = nan', sprintf('wSamples = %d', wSamples));

tempScript = strrep(tempScript, 'offSetW = nan', sprintf('offSetW = %d', wDistance));
tempScript = strrep(tempScript, 'offSetT = nan', sprintf('offSetT = %d', tDistance));

tempScript = strrep(tempScript, 'gainW = nan', sprintf('gainW = %d', gainW));
tempScript = strrep(tempScript, 'gainT = nan', sprintf('gainT = %d', gainT));


tempScript = strrep(tempScript, '//Script name: nan;', sprintf('//Script name: "%s";', saveName));

tempScript = strrep(tempScript, 'std::string fileName = nan;', sprintf('std::string fileName = "%s";', saveName));
tempScript = strrep(tempScript, 'crossOverHz = nan;', sprintf('crossOverHz = %d;', fc));

      if (B_Lo_Length ==3)
          b2_Lo=B_Lo(1,3);
          b2_Hi=B_Hi(1,3);
          a2_Lo=A_Lo(1,3);
          a2_Hi=A_Hi(1,3);

        tempScript = strrep(tempScript, 'a2_Lo = nan', sprintf('a2_Lo = %.31f', a2_Lo));
        tempScript = strrep(tempScript, 'b2_Lo = nan', sprintf('b2_Lo = %.31f', b2_Lo));
        tempScript = strrep(tempScript, 'a2_Hi = nan', sprintf('a2_Hi = %.31f', a2_Hi));
        tempScript = strrep(tempScript, 'b2_Hi = nan', sprintf('b2_Hi = %.31f', b2_Hi));

      elseif (B_Lo_Length ==5)
          b2_Lo=B_Lo(1,3);
          b2_Hi=B_Hi(1,3);
          a2_Lo=A_Lo(1,3);
          a2_Hi=A_Hi(1,3);

          b3_Lo=B_Lo(1,4);
          b3_Hi=B_Hi(1,4);
          a3_Lo=A_Lo(1,4);
          a3_Hi=A_Hi(1,4);

          b4_Lo=B_Lo(1,5);
          b4_Hi=B_Hi(1,5);
          a4_Lo=A_Lo(1,5);
          a4_Hi=A_Hi(1,5);


          
        tempScript = strrep(tempScript, 'a2_Lo = nan', sprintf('a2_Lo = %.31f', a2_Lo));
        tempScript = strrep(tempScript, 'b2_Lo = nan', sprintf('b2_Lo = %.31f', b2_Lo));
        tempScript = strrep(tempScript, 'a2_Hi = nan', sprintf('a2_Hi = %.31f', a2_Hi));
        tempScript = strrep(tempScript, 'b2_Hi = nan', sprintf('b2_Hi = %.31f', b2_Hi));

        tempScript = strrep(tempScript, 'a3_Lo = nan', sprintf('a3_Lo = %.31f', a3_Lo));
        tempScript = strrep(tempScript, 'b3_Lo = nan', sprintf('b3_Lo = %.31f', b3_Lo));
        tempScript = strrep(tempScript, 'a3_Hi = nan', sprintf('a3_Hi = %.31f', a3_Hi));
        tempScript = strrep(tempScript, 'b3_Hi = nan', sprintf('b3_Hi = %.31f', b3_Hi));

        tempScript = strrep(tempScript, 'a4_Lo = nan', sprintf('a4_Lo = %.31f', a4_Lo));
        tempScript = strrep(tempScript, 'b4_Lo = nan', sprintf('b4_Lo = %.31f', b4_Lo));
        tempScript = strrep(tempScript, 'a4_Hi = nan', sprintf('a4_Hi = %.31f', a4_Hi));
        tempScript = strrep(tempScript, 'b4_Hi = nan', sprintf('b4_Hi = %.31f', b4_Hi));

      end

 

% Save modified script to new file
fileID = fopen(saveName, 'w');
disp(['Teensy script saved as:', saveName]);
disp('Loudspeaker Simulation Running...')
fwrite(fileID, tempScript, 'char');


if strcmp(get_param('a_LS_model/Teensy Script', 'saveFigs'),"on")
        
     figSaveFolder = get_param('a_LS_model/Teensy Script', 'figSaveFolder');
     disp(['Figs saved to folder in root: ', figSaveFolder]);

     copyfile(saveName, figSaveFolder);
     disp('Loudspeaker Simulation Running...')

end
fclose(fileID);

flag=2;


end

== matlab function a_LS_model2/Box Modes/Box Modes Function ==
function boxModes()

coder.extrinsic('get_param')
coder.extrinsic('xticks')
coder.extrinsic('xticklabels')
coder.extrinsic('assignin')
coder.extrinsic('evalin')
coder.extrinsic("sgtitle")
coder.extrinsic("exist")
coder.extrinsic("mkdir")
coder.extrinsic("fullfile")
coder.extrinsic("format")
coder.extrinsic("uifigure")
coder.extrinsic("uitable")
coder.extrinsic("uistyle")
coder.extrinsic("uicontrol")
coder.extrinsic("uipanel")
coder.extrinsic("floor")

persistent boxFlag;


depth= str2double(get_param('a_LS_model/Box Modes', 'depth'))*1e-3;
height = str2double(get_param('a_LS_model/Box Modes', 'height'))*1e-3;
width = str2double(get_param('a_LS_model/Box Modes', 'width'))*1e-3;
numberOfModes = 8;
rowNames = cell(numberOfModes,1);

if isempty(boxFlag)
    boxFlag = get_param('a_LS_model/Box Modes', 'boxFlag');
end


    c = 343;
    



    depthModes = ones(numberOfModes,1);
    heightModes = ones(numberOfModes,1);
    widthModes = ones(numberOfModes,1);

    for i=1:numberOfModes
        
        depthModes(i)= floor((c/(2*depth))*i);
        heightModes(i) = floor((c/(2*height))*i);
        widthModes (i) = floor((c/(2*width))*i);         
  
    end
    

    cNames = {'Depth'; 'Height'; 'Width'};
   

    modes = [depthModes, heightModes, widthModes];
    found=zeros(size(modes));
    toFind=double(0);
    
    %loop through matrix to find duplicates
    
    for m=1:3
        for j =1:numberOfModes
            toFind=modes(j,m); 
            for n=1:3
                for i=int8(1):numberOfModes
                    if modes(i, n) == toFind && (i ~= j && n ~= m)
                        found(i,n) = modes(i,n);
                        
                    end
                end
            end
        
        end
    
    end
    

    for i =int8(1):numberOfModes
            
        rowNames {i} = sprintf('Mode %d\n (Hz)',i);
    
    end

     

    if strcmp(boxFlag, 'on')
    figure(12)
    panel1 = uipanel('Title', 'Box Modes', 'TitlePosition','centertop','Position', [0.05, 0.05, 0.5, 0.9], 'FontSize', 18,'BackgroundColor', '#FFFDD0');
    panel2 = uipanel('Title', 'Duplicate Modes','TitlePosition','centertop', 'Position', [0.55, 0.05, 0.4, 0.9],'FontSize', 18, 'BackgroundColor', '#FFFDD0');
    
    uitable(panel1,"Data",modes, "ColumnName",cNames, 'RowName', rowNames,'Units', 'normalized','FontSize', 18);
    

       
    data = found;

    uitable(panel2, 'Data', data, "ColumnName",cNames,'RowName',rowNames, 'Units', 'normalized','FontSize', 18);

   set(gcf,'Position',[10 10 1000 400])

   if strcmp(get_param('a_LS_model/Teensy Script', 'saveFigs'),"on")
            
       figSaveFolder = get_param('a_LS_model/Teensy Script', 'figSaveFolder');
            
            
            if ~exist(figSaveFolder, 'dir')
                
                mkdir(figSaveFolder);
            
            end
            
            saveas(gcf,fullfile(figSaveFolder,[figSaveFolder,'_boxModes.png']));
            
     end
        
   end

    
    
    boxFlag = 'off';


end

== matlab function a_LS_model2/Subsystem5/MATLAB Function ==
  data: f_out output; x input

function f_out=variableResistor(x)

coder.extrinsic('get_param')


persistent endIndex
persistent t
persistent f f_padded
persistent N
persistent SweepStart SweepDuration SweepStop fs xLength




if isempty(t)
    endIndex=1;
    xLength=length(x);
    
    SweepDuration=double(0);
    SweepStart =str2double(get_param('a_LS_model/Subsystem4', 'SweepStart'));
    SweepStop = str2double(get_param('a_LS_model/Subsystem4', 'SweepStop'));
    SweepDuration =str2double(get_param('a_LS_model/Subsystem4', 'SweepTime'));

    fs=44100;

    t = 0:1/fs:SweepDuration-1/fs;
    N=numel(t);
    f = logspace(log10(SweepStart),log10(SweepStop),N);
    pad_length = 1024 - mod(N, 1024);  % Calculate the number of elements to pad at the end
    f_padded = [f'; ones(pad_length, 1)];  % pad the end of f
    f_out = zeros(size(x));

end


        
f_out = f_padded(endIndex:endIndex+xLength-1);

endIndex=endIndex+xLength;


%%
%%%%%%%%%%%%%%%%%%%%%%%%%%%%%%%%%%%%%%%%%%%%%%%%%%%%%%%%%%%%%%%%%%%%%%%%%%%%%%%%%%%%%%%%%%%%%%%%%%%%%%%%%%%%%%%%%%%%%%%%%%%%%%%%%%%%





end
